simulink model "Subsystem"  (R2020b)
settings: Solver=FixedStepAuto  StartTime=0.0  StopTime=10.0  FixedStep=0.2  RelTol=1e-3
values from neighbouring files (symbols this model uses):
  a0 = 1.0    [Data_dict.sldd]
  a1 = 2.0    [Data_dict.sldd]
  a2 = -3.0    [Data_dict.sldd]
  a3 = -4.0    [Data_dict.sldd]
  a4 = 5.0    [Data_dict.sldd]
settings Model: DataDictionary=Data_dict.sldd  Creator=Shree  LastModifiedBy=Shree
settings DataIOCC: SaveOutput=off  SaveTime=off

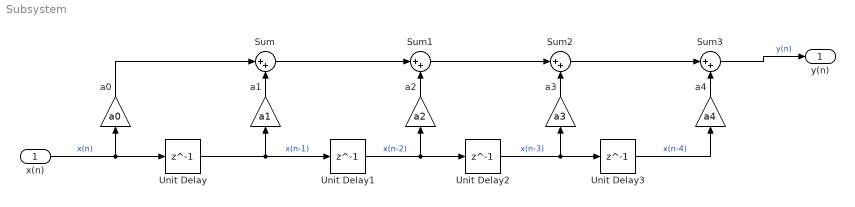
== system Subsystem ==
  x(n) : Inport  OutDataTypeStr=double  PortDimensions=1  SampleTime=[0.20000000000000001,0]
  " Unit Delay" : Delay  DelayLength=1  InitialCondition=0
  " Unit Delay1" : Delay  DelayLength=1  InitialCondition=0
  Sum{,1..3} (4 alike) : Sum  Inputs=|++
  Unit Delay2 : Delay  DelayLength=1  InitialCondition=0
  Unit Delay3 : Delay  DelayLength=1  InitialCondition=0
  a0 : Gain  Gain=a0
  a1 : Gain  Gain=a1
  a2 : Gain  Gain=a2
  a3 : Gain  Gain=a3
  a4 : Gain  Gain=a4
  y(n) : Outport  OutDataTypeStr=double  PortDimensions=1  SampleTime=[0.20000000000000001,0]
  wires:
  " Unit Delay1"/1 -> Unit Delay2/1, a2/1  "x(n-2)"
  a2/1 -> Sum1/2
  x(n)/1 -> a0/1, " Unit Delay"/1  "x(n)"
  a4/1 -> Sum3/2
  Sum2/1 -> Sum3/1
  a0/1 -> Sum/1
  a3/1 -> Sum2/2
  a1/1 -> Sum/2
  Unit Delay3/1 -> a4/1  "x(n-4)"
  Sum1/1 -> Sum2/1
  Sum/1 -> Sum1/1
  Unit Delay2/1 -> Unit Delay3/1, a3/1  "x(n-3)"
  " Unit Delay"/1 -> " Unit Delay1"/1, a1/1  "x(n-1)"
  Sum3/1 -> y(n)/1  "y(n)"
